simulink model "filtroduplo"  (R2021b)
settings: Solver=FixedStepDiscrete  StartTime=0.0  StopTime=600  FixedStep=0.1  RelTol=1e-3  AbsTol=1e-3  EnableMultiTasking=on
libraries: fl_lib x7, nesl_utility x4, ee_lib x2, raspberrypiCommlib x2, slrealtimeseriallib x1
settings Model: Creator=Pc melhor q do euler  LastModifiedBy=Pc melhor q do euler
settings SolverCC: AutoScaleAbsTol=off  AlgebraicLoopSolver=TrustRegion  PositivePriorityOrder=on
settings OptimizationCC: UseDivisionForNetSlopeComputation=on  GainParamInheritBuiltInType=on  UseFloatMulNetSlope=on  EnhancedBackFolding=on  PassReuseOutputArgsAs=Individual arguments  ZeroExternalMemoryAtStartup=off  ZeroInternalMemoryAtStartup=off  EfficientFloat2IntCast=on  MaxStackSize=64  OptimizeBlockOrder=speed  DifferentSizesBufferReuse=on  OptimizationCustomize=off  EfficientTunableParamExpr=on
settings DebuggingCC: ParameterTunabilityLossMsg=error  SymbolicDimsDataTypeCodeGenerationDiagnostic=none  SFMachineParentedDataDiag=warning
settings HardwareCC: ProdBitPerPointer=32  ProdBitPerSizeT=32  ProdBitPerPtrDiffT=32  ProdLargestAtomicInteger=Long  ProdLargestAtomicFloat=Double  ProdWordSize=32  ProdLongLongMode=on  ProdHWDeviceType=ARM Compatible->ARM Cortex
settings SFSimCC: CustomCodeUndefinedFunction=UseInterfaceOnly
settings RTWCC: Description=Embedded Coder  SystemTargetFile=ert.tlc  HardwareBoard=Raspberry Pi  TLCOptions="-aInlineSetEventsForThisBaseRateFcn=TLC_FALSE -aSuppressMultiTaskScheduler=TLC_FALSE  -aRateBasedStepFcn=0"  TemplateMakefile=ert_default_tmf  Toolchain=GNU GCC Embedded Linux  BuildConfiguration=Faster Runs  CheckMdlBeforeBuild=Warning
settings CodeAppCC: ForceParamTrailComments=on  IgnoreCustomStorageClasses=off  OperatorAnnotations=on  SimulinkDataObjDesc=on  SFDataObjDesc=on  InsertBlockDesc=on
settings ERTTargetCC: SupportContinuousTime=on  SupportVariableSizeSignals=on  ExtModeStaticAlloc=on
settings SimscapeCC: EditingMode=Restricted  SimscapeNormalizeSystem=off  SimscapeLogSimulationStatistics=on  SimscapeLogDataHistory=10000

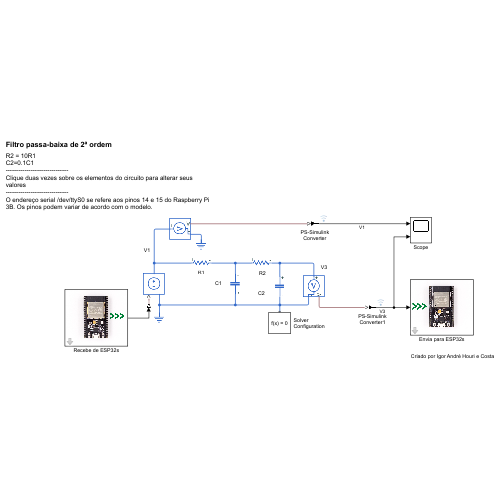
[thumbnail: Simulink's stored preview of the top-level diagram]
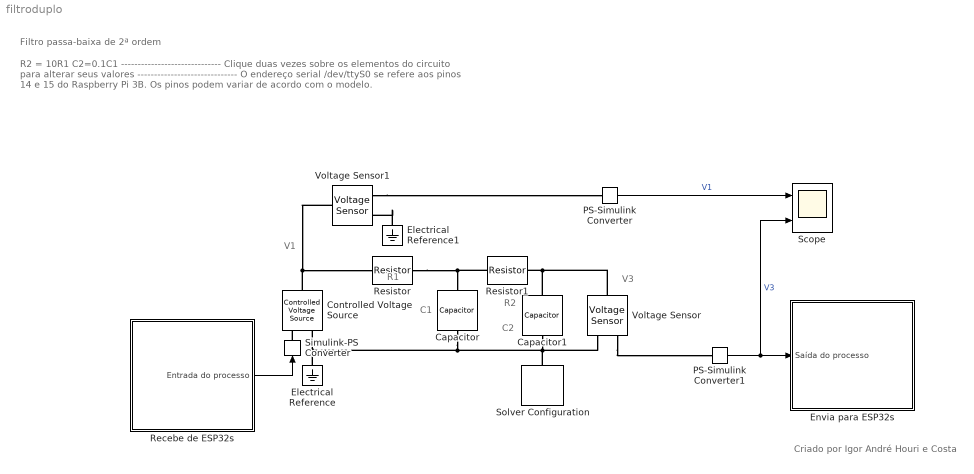
== system filtroduplo ==
  note: Criado por Igor André Houri e Costa
  note: V3
  note: V1
  note: C1
  note: R1
  note: R2 = 10R1
      | C2=0.1C1
      | ------------------------------
      | Clique duas vezes sobre os elementos do circuito para alterar seus valores
      | ------------------------------
      | O endereço serial /dev/ttyS0 se refere aos pinos 14 e 15 do Raspberry Pi 3B. Os pinos podem variar de acordo com o modelo.
  note: Filtro passa-baixa de 2ª ordem
  note: R2
  note: C2
  Capacitor : ee_lib/Passive/Capacitor  cap_option=0  c=0.016 F  Cvec=[1e-05, 1e-06] F  Vvec=[0, 10] V  CV_table_symmetry=1  f_vec=[1, 10] kHz  DFext_vec=[.8, 1.2]  C_tol=5  enable_C_tol=0  tol_distribution=1  nSigma=4  r=1e-6 Ohm  g=0 1/Ohm  averaging_period=0 s  enable_operating_limits=0  operating_limit_action=2  max_working_voltage_range=[-25, 25] V  power_rating=1 W  enable_faults=0  fault_action=1  Cscale_faulted=100  R_faulted=1e-3 Ohm  G_faulted=0 1/Ohm  tau_fault=1e-3 s  enable_temporal_fault=0  t_fault=1 s  enable_behavioral_fault=0  max_permissible_voltage_range=[-100, 100] V  t_fail_on_voltage=1 s  i_specify=off  i_priority=None  i=0 A  i_nominal_specify=off  i_nominal_unit=A  i_nominal_value=1  v_specify=off  v_priority=None  v=0 V  v_nominal_specify=off  v_nominal_unit=V  v_nominal_value=1  vc_specify=off  vc_priority=High  vc=0 V  vc_nominal_specify=off  vc_nominal_unit=V  vc_nominal_value=1
  Capacitor1 : ee_lib/Passive/Capacitor  cap_option=0  c=0.0016 F  Cvec=[1e-05, 1e-06] F  Vvec=[0, 10] V  CV_table_symmetry=1  f_vec=[1, 10] kHz  DFext_vec=[.8, 1.2]  C_tol=5  enable_C_tol=0  tol_distribution=1  nSigma=4  r=1e-6 Ohm  g=0 1/Ohm  averaging_period=0 s  enable_operating_limits=0  operating_limit_action=2  max_working_voltage_range=[-25, 25] V  power_rating=1 W  enable_faults=0  fault_action=1  Cscale_faulted=100  R_faulted=1e-3 Ohm  G_faulted=0 1/Ohm  tau_fault=1e-3 s  enable_temporal_fault=0  t_fault=1 s  enable_behavioral_fault=0  max_permissible_voltage_range=[-100, 100] V  t_fail_on_voltage=1 s  i_specify=off  i_priority=None  i=0 A  i_nominal_specify=off  i_nominal_unit=A  i_nominal_value=1  v_specify=off  v_priority=None  v=0 V  v_nominal_specify=off  v_nominal_unit=V  v_nominal_value=1  vc_specify=off  vc_priority=High  vc=0 V  vc_nominal_specify=off  vc_nominal_unit=V  vc_nominal_value=1
  Controlled Voltage Source : fl_lib/Electrical/Electrical Sources/Controlled Voltage Source
  Electrical Reference : fl_lib/Electrical/Electrical Elements/Electrical Reference
  Electrical Reference1 : fl_lib/Electrical/Electrical Elements/Electrical Reference
  Envia para ESP32s : Subsystem  mask(Envio de mensagem Serial - ESP32s){board=Pi 3 Model B, SCIModule_=/dev/ttyS0, Baudrate_=115200, Saida_maxima=15, Saida_minima=0}
      mask prompts: SCIModule_ "Port:"; Baudrate_ "Baudrate (in bits/s):"; Saida_maxima "Saída máxima do processo"; Saida_minima "Saída mínima do processo"
      mask help: Este bloco recebe em sua entrada um sinal do tipo double, converte-o para a escala necessária e a envia, via mensagem serial, para o ESP32s. --Bloco criado por Igor Costa.
      mask TypeOptions board: Serial Write/board
      mask TypeOptions SCIModule_: Serial Write/SCIModule_
      mask TypeOptions Baudrate_: Serial Write/Baudrate_
      mask TypeOptions Saida_maxima: Função Map (saída)/Saida_maxima
      mask TypeOptions Saida_minima: Função Map (saída)/Saida_minima
      mask Display: image('$imagefile'); % Use "Edit Image" on toolstrip to change.
  PS-Simulink Converter : nesl_utility/PS-Simulink Converter  PhysicalDomain=network_engine_domain  SubClassName=ps_output  LeftPortType=input  RightPortType=output  PseudoPeriodic=off  Frequencies=[]  Unit=inherit  AffineConversion=off
      settings: SourceProductBaseCode=PW,SS
  PS-Simulink Converter1 : nesl_utility/PS-Simulink Converter  PhysicalDomain=network_engine_domain  SubClassName=ps_output  LeftPortType=input  RightPortType=output  PseudoPeriodic=off  Frequencies=[]  Unit=inherit  AffineConversion=off
      settings: SourceProductBaseCode=PW,SS
  Recebe de ESP32s : Subsystem  mask(Recepção de mensagem Serial - ESP32s){board=Pi 3 Model B, SCIModule_=/dev/ttyS0, Baudrate_=115200, entrada_maxima=15, entrada_minima=0}
      mask prompts: SCIModule_ "Port:"; Baudrate_ "Baudrate (in bits/s):"; entrada_maxima "Entrada máxima do processo"; entrada_minima "Entrada mínima do processo"
      mask help: Este bloco recebe a mensagem serial enviada pelo ESP32s, decodifica-a e converte para a escala configurada; disponibilizando o resultado em sua saída. --Bloco criado por Igor Costa.
      mask TypeOptions board: Serial Read1/board
      mask TypeOptions SCIModule_: Serial Read1/SCIModule_
      mask TypeOptions Baudrate_: Serial Read1/Baudrate_
      mask TypeOptions entrada_maxima: Função Map (entrada)/entrada_maxima
      mask TypeOptions entrada_minima: Função Map (entrada)/entrada_minima
      mask Display: image('I:\PFC_Igor\plot figuras\figuras\Recebe de ESP32s.png'); % Use "Edit Image" on toolstrip to change.
  Resistor : fl_lib/Electrical/Electrical Elements/Resistor  R=1000 Ohm  i_specify=off  i_priority=None  i=0 A  i_nominal_specify=off  i_nominal_unit=A  i_nominal_value=1  v_specify=off  v_priority=None  v=0 V  v_nominal_specify=off  v_nominal_unit=V  v_nominal_value=1
  Resistor1 : fl_lib/Electrical/Electrical Elements/Resistor  R=10000 Ohm  i_specify=off  i_priority=None  i=0 A  i_nominal_specify=off  i_nominal_unit=A  i_nominal_value=1  v_specify=off  v_priority=None  v=0 V  v_nominal_specify=off  v_nominal_unit=V  v_nominal_value=1
  Scope : Scope  NumInputPorts=2
  Simulink-PS Converter : nesl_utility/Simulink-PS Converter  PhysicalDomain=network_engine_domain  SubClassName=ps_input  LeftPortType=input  RightPortType=output  PseudoPeriodic=off  Frequencies=[]  NoiseDistribution=none  NoiseParameters=[]  Unit=1  AffineConversion=off  FilteringAndDerivatives=provide  SimscapeFilterOrder=1  InputFilterTimeConstant=0.001  UdotUserProvided=0
      settings: SourceProductBaseCode=PW,SS
  Solver Configuration : nesl_utility/Solver Configuration  PhysicalDomain=network_engine_domain  SubClassName=solver  LeftPortType=input  RightPortType=generic  Tones=[]  Harmonics=[]  SimulateNoise=off  Profile=off  UseLocalSampling=off  EnableSwitchedLinearOptims=on  FrequencyDomain=off  UseCCode=off  RelTol=0.001  AbsTol=1e-06  MinStep=1e-09  ToWorkspace=off  RevertToSquareIcSolve=off  NumHomotopyIterations=100  PhasorMode=off  PhasorModeNumHarmonics=1  DoDC=off  ResidualTolerance=1e-09  UseLocalSolver=on  LocalSolverChoice=NE_TRAPEZOIDAL_ADVANCER  LocalSolverSampleTime=0.1  DoFixedCost=on  MaxNonlinIter=3  MaxModeIter=2  ComputeImpulses=off  ImpulseIterations=2  LinearAlgebra=auto  EquationFormulation=NE_TIME_EF  DelaysMemoryBudget=1024  AutomaticFiltering=on  FilteringTimeConstant=0.001  PartitionStorageMethod=AS_NEEDED  PartitionMemoryBudget=1024  PartitionMethod=ROBUST
      settings: SourceProductBaseCode=PW,SS
  Voltage Sensor : fl_lib/Electrical/Electrical Sensors/Voltage Sensor
  Voltage Sensor1 : fl_lib/Electrical/Electrical Sensors/Voltage Sensor
  wires:
  PS-Simulink Converter/1 -> Scope/1  "V1"
  PS-Simulink Converter1/1 -> Scope/2, Envia para ESP32s/1(Saída do processo)  "V3"
  Recebe de ESP32s/1(Entrada do processo) -> Simulink-PS Converter/1
  connections:
  Resistor/RConn1 -- Resistor1/LConn1 -- Capacitor/LConn1
  Solver Configuration/RConn1 -- Voltage Sensor/RConn2 -- Capacitor1/RConn1 -- Capacitor/RConn1 -- Electrical Reference/LConn1 -- Controlled Voltage Source/RConn2
  Controlled Voltage Source/LConn1 -- Voltage Sensor1/LConn1 -- Resistor/LConn1
  Capacitor1/LConn1 -- Voltage Sensor/LConn1 -- Resistor1/RConn1
  Simulink-PS Converter/RConn1 -- Controlled Voltage Source/RConn1
  Voltage Sensor/RConn1 -- PS-Simulink Converter1/LConn1
  Voltage Sensor1/RConn1 -- PS-Simulink Converter/LConn1
  Electrical Reference1/LConn1 -- Voltage Sensor1/RConn2

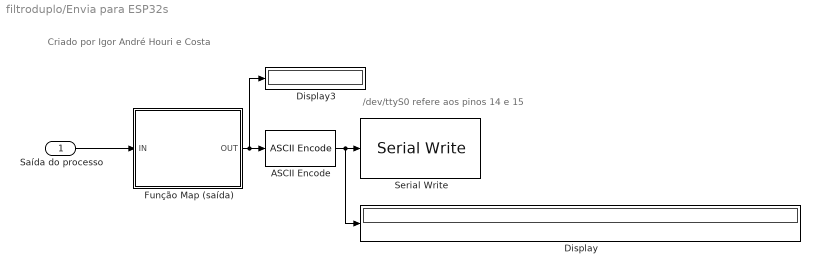
== system filtroduplo/Envia para ESP32s ==
  note: /dev/ttyS0 refere aos pinos 14 e 15
  note: Criado por Igor André Houri e Costa
  Saída do processo : Inport
  ASCII Encode : slrealtimeseriallib/ASCII Encode  format=%d\r  nvars=1  maxlength=32  vartypes={ 'double' }
      settings: SourceProductBaseCode=XP
  Display : Display
  Display3 : Display
  Função Map (saída) : Subsystem  mask(Função Map - entrada){Saida_maxima=Saida_maxima, Saida_minima=Saida_minima}
      mask prompts: Saida_maxima "Saída máxima do processo"; Saida_minima "Saída mínima do processo"
      mask help: Este bloco mapeia um número de uma escala (range) para a escala necessária para envio da saída do processo ao ESP32s (0 a 4095). A função implementada é (x - x_min) * (4095 - 0) / (x_max - x_min) + 0, sendo "x" o valor do número a ser mapeado, "x_min" o menor valor possível para x e "x_max" o maior valor possível para x. --Bloco criado por Igor Costa.
      mask Help: sdsd
      mask TypeOptions Saida_maxima: Saida_maxima/Value
      mask TypeOptions Saida_minima: Saida_minima/Value
  Serial Write : raspberrypiCommlib/Serial Write  board=Pi 3 Model B  SCIModule_=/dev/ttyS0  Baudrate_=115200  Parity=None  StopBits_=1  HardwareFlowControl=None  ByteOrder=LittleEndian  OutputStatus=off  blockPlatform=RaspberryPi
      settings: SourceProductBaseCode=RASPPI
  wires:
  Função Map (saída)/1(OUT) -> Display3/1, ASCII Encode/1
  ASCII Encode/1 -> Display/1, Serial Write/1
  Saída do processo/1 -> Função Map (saída)/1(IN)

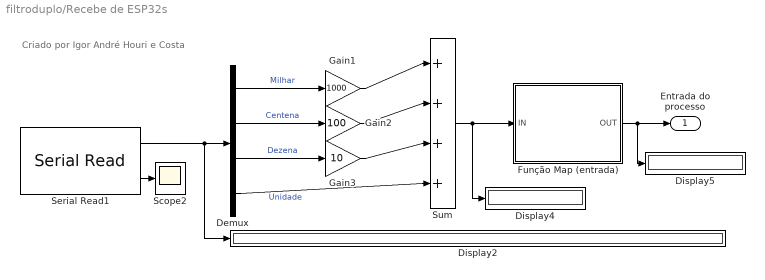
== system filtroduplo/Recebe de ESP32s ==
  note: Criado por Igor André Houri e Costa
  Demux : Demux
  Display2 : Display
  Display4 : Display
  Display5 : Display
  Função Map (entrada) : Subsystem  mask(Função Map - entrada){entrada_maxima=entrada_maxima, entrada_minima=entrada_minima}
      mask prompts: entrada_maxima "Entrada máxima do processo"; entrada_minima "Entrada mínima do processo"
      mask help: Este bloco mapeia um número de uma escala (range) da escala necessária para decodificação da entrada do processo recebida ESP32s (0 a 4095), passando-o para a escala dos valores do processo. A função implementada é (x - 0) * (x_max - x_min) / (4095 - 0), sendo "x" o valor do número a ser mapeado, "x_min" o menor valor possível para x e "x_max" o maior valor possível para x. --Bloco criado por Igor Costa.
      mask TypeOptions entrada_maxima: Entrada_maxima/Value
      mask TypeOptions entrada_minima: Entrada_minima/Value
  Gain1 : Gain  Gain=1000
  Gain2 : Gain  Gain=100
  Gain3 : Gain  Gain=10
  Scope2 : Scope
  Serial Read1 : raspberrypiCommlib/Serial Read  board=Pi 3 Model B  SCIModule_=/dev/ttyS0  Baudrate_=115200  Parity=None  StopBits_=1  HardwareFlowControl=None  ByteOrder=LittleEndian  DataLength=4  DataType=uint8  OutputStatus=on  SampleTime=0.1  blockPlatform=RaspberryPi
      settings: SourceProductBaseCode=RASPPI
  Sum : Sum  Inputs=|++++
  Entrada do processo : Outport
  wires:
  Demux/3 -> Gain3/1  "Dezena"
  Demux/4 -> Sum/4  "Unidade"
  Demux/2 -> Gain2/1  "Centena"
  Serial Read1/2 -> Scope2/1
  Demux/1 -> Gain1/1  "Milhar"
  Sum/1 -> Display4/1, Função Map (entrada)/1(IN)
  Gain1/1 -> Sum/1
  Gain2/1 -> Sum/2
  Serial Read1/1 -> Display2/1, Demux/1
  Gain3/1 -> Sum/3
  Função Map (entrada)/1(OUT) -> Display5/1, Entrada do processo/1

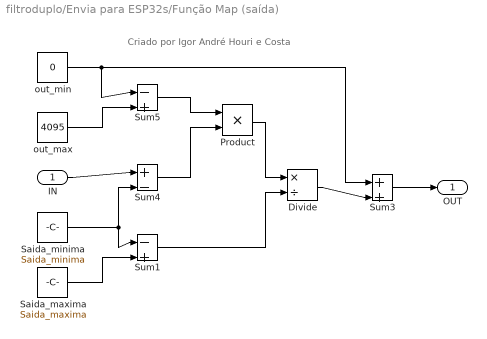
== system filtroduplo/Envia para ESP32s/Função Map (saída) ==
  note: Criado por Igor André Houri e Costa
  IN : Inport
  Divide : Product  Inputs=*/
  Product : Product
  Saida_maxima : Constant  Value=Saida_maxima
  Saida_minima : Constant  Value=Saida_minima
  Sum1 : Sum  Inputs=|-+
  Sum3 : Sum  Inputs=++|
  Sum4 : Sum  Inputs=|+-
  Sum5 : Sum  Inputs=|-+
  out_max : Constant  Value=4095
  out_min : Constant  Value=0
  OUT : Outport
  wires:
  Sum5/1 -> Product/1
  out_max/1 -> Sum5/2
  Sum1/1 -> Divide/2
  Saida_minima/1 -> Sum4/2, Sum1/1
  IN/1 -> Sum4/1
  out_min/1 -> Sum3/1, Sum5/1
  Divide/1 -> Sum3/2
  Sum4/1 -> Product/2
  Product/1 -> Divide/1
  Sum3/1 -> OUT/1
  Saida_maxima/1 -> Sum1/2

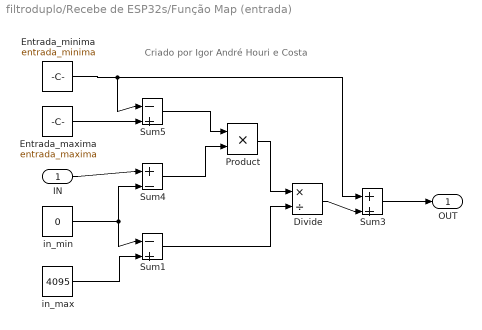
== system filtroduplo/Recebe de ESP32s/Função Map (entrada) ==
  note: Criado por Igor André Houri e Costa
  IN : Inport
  Divide : Product  Inputs=*/
  Entrada_maxima : Constant  Value=entrada_maxima
  Entrada_minima : Constant  Value=entrada_minima
  Product : Product
  Sum1 : Sum  Inputs=|-+
  Sum3 : Sum  Inputs=++|
  Sum4 : Sum  Inputs=|+-
  Sum5 : Sum  Inputs=|-+
  in_max : Constant  Value=4095
  in_min : Constant  Value=0
  OUT : Outport
  wires:
  Sum5/1 -> Product/1
  Sum1/1 -> Divide/2
  IN/1 -> Sum4/1
  Entrada_minima/1 -> Sum3/1, Sum5/1
  Divide/1 -> Sum3/2
  Sum4/1 -> Product/2
  Product/1 -> Divide/1
  Sum3/1 -> OUT/1
  in_max/1 -> Sum1/2
  in_min/1 -> Sum1/1, Sum4/2
  Entrada_maxima/1 -> Sum5/2
